simulink model "GlucoseModel2016b"  (R2016b)
settings: Solver=ode4  StartTime=0.0  StopTime=371  FixedStep=.1  RelTol=1e-3  EnableMultiTasking=on
values from neighbouring files (symbols this model uses):
  Bio = min(sqrt(120*12)*rand() + 50, 87) / 100    [GlucoseModelInit.m]
  EGP_0 = lognrnd(log(.0169), .86) * kg    [GlucoseModelInit.m]
  Fs_01 = 11.1 * 10^-3 * kg    (= 0.999)    [GlucoseModelInit.m]
  G_1_0 = 0    [GlucoseModelInit.m]
  G_2_0 = 0    [GlucoseModelInit.m]
  I_0 = 1.15    [GlucoseModelInit.m]
  k_12 = max(min(lognrnd(-2.813, .43), .2), .01)    [GlucoseModelInit.m]
  k_a = max(min(normrnd(.018, .0045), .06), .005)    [GlucoseModelInit.m]
  k_a_int = lognrnd(-2.372, 1.092)    [GlucoseModelInit.m]
  k_b1 = max(min(lognrnd(-5.684, 1.00), .05), .0002)    [GlucoseModelInit.m]
  k_b2 = max(min(lognrnd(-2.882, .75), .4), .005)    [GlucoseModelInit.m]
  k_b3 = max(min(lognrnd(-3.730, .75), .1), .003)    [GlucoseModelInit.m]
  k_e = max(min(normrnd(.14, .0345), .3), .05)    [GlucoseModelInit.m]
  Q_1_0 = G_0 * V_G    (= 203.51601)    [GlucoseModelInit.m]
  R_cl = max(min(normrnd(.01, .025), .03), .003)    [GlucoseModelInit.m]
  R_thr = max(min(normrnd(9, 1.5), 15.0), 7.5)    [GlucoseModelInit.m]
  S_1_0 = 0    [GlucoseModelInit.m]
  S_2_0 = 0    [GlucoseModelInit.m]
  S_ID = 1.58 * 10^-4    (= 0.000158)    [GlucoseModelInit.m]
  S_IE = 73 * 10^-4    (= 0.0073)    [GlucoseModelInit.m]
  S_IT = 11.0 * 10^-4    (= 0.0011)    [GlucoseModelInit.m]
  t_max = 1 / max(min(lognrnd(-3.689, 0.252), .035), .02)    [GlucoseModelInit.m]
  V_G = max(min(lognrnd(-1.897, .23), .25), .09) * kg    [GlucoseModelInit.m]
  V_I = max(min(normrnd(.12, .012), .18), .08) * kg    [GlucoseModelInit.m]
settings Model: Creator=brier245  LastModifiedBy=aegawe01
settings SolverCC: ZeroCrossControl=DisableAll
settings DataIOCC: SaveFormat=Structure  ReturnWorkspaceOutputs=on  ReturnWorkspaceOutputsName=SDOSimTest_Log
settings OptimizationCC: LifeSpan=inf
settings DebuggingCC: SFUnexpectedBacktrackingDiag=warning  SFNoUnconditionalDefaultTransitionDiag=warning  SFExecutionAtInitializationDiag=none
settings HardwareCC: ProdBitPerPointer=32  ProdBitPerSizeT=32  ProdBitPerPtrDiffT=32  ProdLargestAtomicFloat=None  ProdIntDivRoundTo=Undefined  ProdEndianess=Unspecified  ProdWordSize=32  ProdHWDeviceType=32-bit Generic
settings ModelReferenceCC: PropagateSignalLabelsOutOfModel=off
settings GRTTargetCC: TargetLangStandard=C89/C90 (ANSI)  GeneratePreprocessorConditionals=Disable all
settings ConfigComp: CovMetricSettings=dw  CovHtmlReporting=on  CovSaveCumulativeToWorkspaceVar=on  CovSaveSingleToWorkspaceVar=on  CovExternalEMLEnable=off

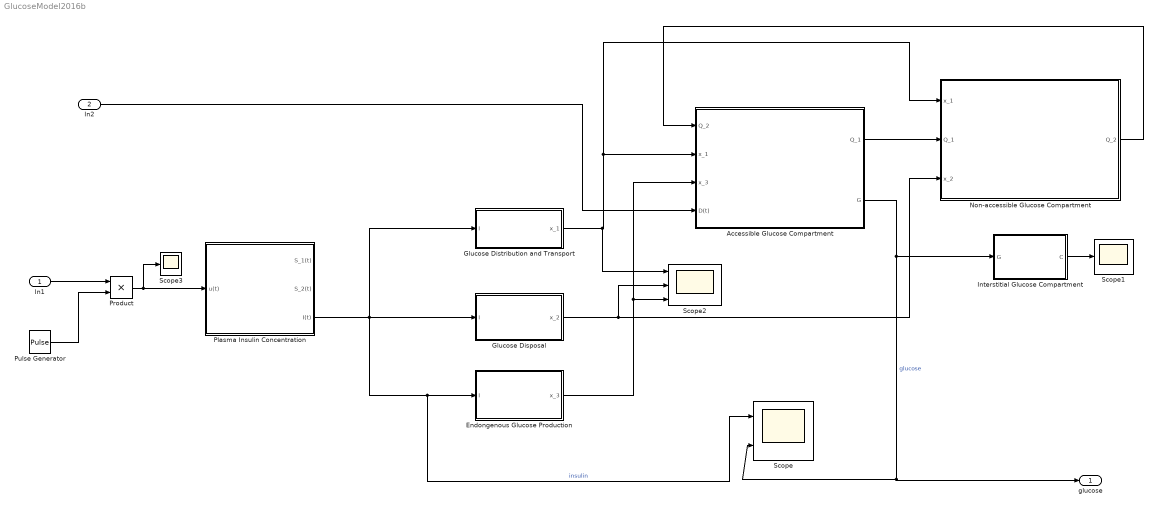
== system GlucoseModel2016b ==
  In1 : Inport
  In2 : Inport  Port=2
  Accessible Glucose Compartment : Subsystem
  Endongenous Glucose Production : Subsystem
  Glucose Disposal : Subsystem
  Glucose Distribution and Transport : Subsystem
  Interstitial Glucose Compartment : Subsystem
  Non-accessible Glucose Compartment : Subsystem
  Plasma Insulin Concentration : Subsystem
  Product : Product
  Pulse Generator : DiscretePulseGenerator  PulseType=Time based  Period=60  PulseWidth=100./60
  Scope : Scope  NumInputPorts=2
  Scope1 : Scope
  Scope2 : Scope  NumInputPorts=3
  Scope3 : Scope
  glucose : Outport
  wires:
  Accessible Glucose Compartment/1(Q_1) -> Non-accessible Glucose Compartment/2(Q_1)
  Non-accessible Glucose Compartment/1(Q_2) -> Accessible Glucose Compartment/1(Q_2)
  Plasma Insulin Concentration/3(I(t)) -> Glucose Distribution and Transport/1(I), Glucose Disposal/1(I), Scope/1, Endongenous Glucose Production/1(I)  "insulin"
  Glucose Distribution and Transport/1(x_1) -> Scope2/1, Accessible Glucose Compartment/2(x_1), Non-accessible Glucose Compartment/1(x_1)
  Glucose Disposal/1(x_2) -> Scope2/2, Non-accessible Glucose Compartment/3(x_2)
  Endongenous Glucose Production/1(x_3) -> Accessible Glucose Compartment/3(x_3), Scope2/3
  Accessible Glucose Compartment/2(G) -> glucose/1, Scope/2, Interstitial Glucose Compartment/1(G)  "glucose"
  Interstitial Glucose Compartment/1(C) -> Scope1/1
  In2/1 -> Accessible Glucose Compartment/4(D(t))
  In1/1 -> Product/1
  Pulse Generator/1 -> Product/2
  Product/1 -> Scope3/1, Plasma Insulin Concentration/1(u(t))

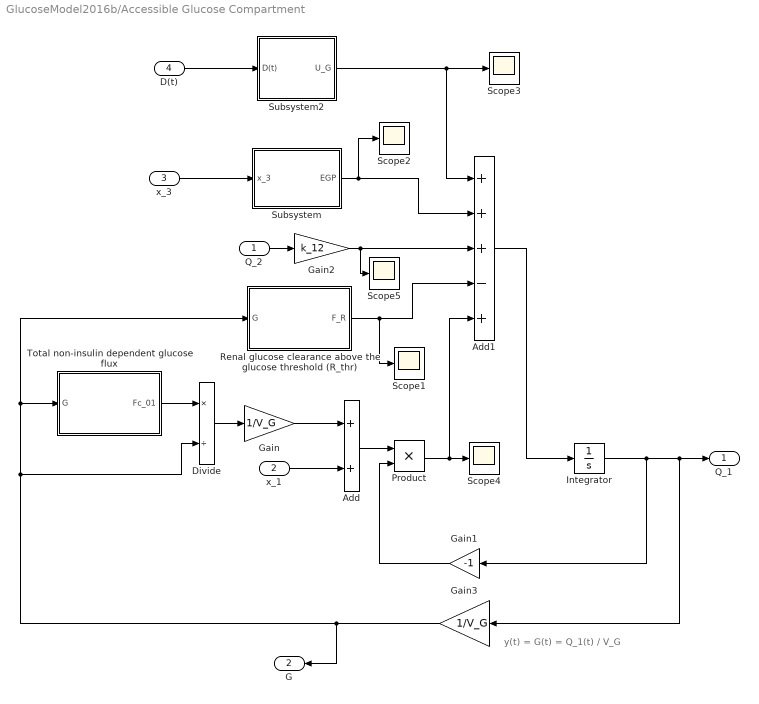
== system GlucoseModel2016b/Accessible Glucose Compartment ==
  note: y(t) = G(t) = Q_1(t) / V_G
  Q_2 : Inport
  x_1 : Inport  Port=2
  x_3 : Inport  Port=3
  D(t) : Inport  Port=4
  Add : Sum
  Add1 : Sum  Inputs=+++-+
  Divide : Product  Inputs=*/
  Gain : Gain  Gain=1/V_G
  Gain1 : Gain  Gain=-1
  Gain2 : Gain  Gain=k_12
  Gain3 : Gain  Gain=1/V_G
  Integrator : Integrator  InitialCondition=Q_1_0  LimitOutput=on  LowerSaturationLimit=0
  Product : Product
  Renal glucose clearance above the glucose threshold (R_thr) : Subsystem
  Scope{1..5} (5 alike) : Scope
  Subsystem : Subsystem
  Subsystem2 : Subsystem
  Total non-insulin dependent glucose flux : Subsystem
  Q_1 : Outport
  G : Outport  Port=2
  wires:
  x_1/1 -> Add/2
  Q_2/1 -> Gain2/1
  Product/1 -> Scope4/1, Add1/5
  Total non-insulin dependent glucose flux/1(Fc_01) -> Divide/1
  Divide/1 -> Gain/1
  Integrator/1 -> Gain3/1, Q_1/1, Gain1/1
  Add1/1 -> Integrator/1
  x_3/1 -> Subsystem/1(x_3)
  Gain1/1 -> Product/2
  Renal glucose clearance above the glucose threshold (R_thr)/1(F_R) -> Scope1/1, Add1/4
  Subsystem/1(EGP) -> Scope2/1, Add1/2
  Gain/1 -> Add/1
  Add/1 -> Product/1
  Gain2/1 -> Scope5/1, Add1/3
  D(t)/1 -> Subsystem2/1(D(t))
  Subsystem2/1(U_G) -> Add1/1, Scope3/1
  Gain3/1 -> G/1, Divide/2, Renal glucose clearance above the glucose threshold (R_thr)/1(G), Total non-insulin dependent glucose flux/1(G)

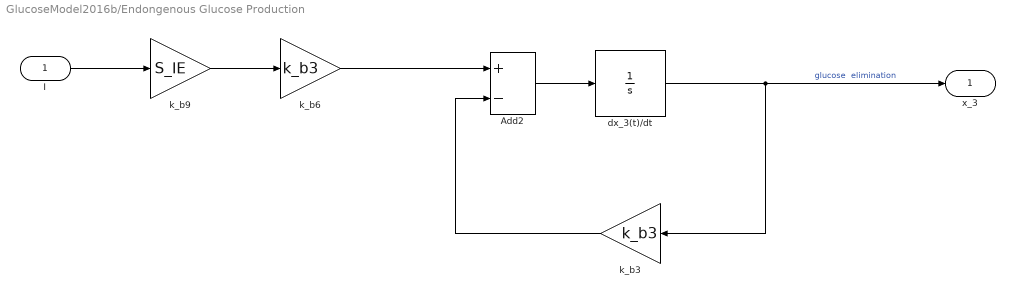
== system GlucoseModel2016b/Endongenous Glucose Production ==
  I : Inport
  Add2 : Sum  Inputs=+-
  dx_3(t)/dt : Integrator  InitialCondition=S_IE*I_0  LimitOutput=on  LowerSaturationLimit=0
  k_b3 : Gain  Gain=k_b3
  k_b6 : Gain  Gain=k_b3
  k_b9 : Gain  Gain=S_IE
  x_3 : Outport
  wires:
  k_b9/1 -> k_b6/1
  dx_3(t)/dt/1 -> x_3/1, k_b3/1  "glucose  elimination"
  Add2/1 -> dx_3(t)/dt/1
  k_b3/1 -> Add2/2
  k_b6/1 -> Add2/1
  I/1 -> k_b9/1

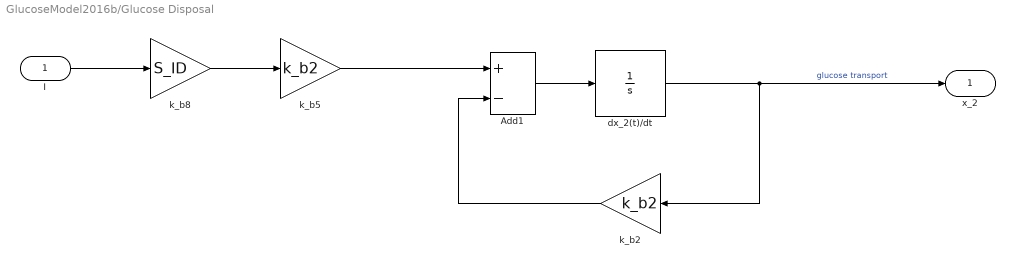
== system GlucoseModel2016b/Glucose Disposal ==
  I : Inport
  Add1 : Sum  Inputs=+-
  dx_2(t)/dt : Integrator  InitialCondition=S_ID*I_0  LimitOutput=on  LowerSaturationLimit=0
  k_b2 : Gain  Gain=k_b2
  k_b5 : Gain  Gain=k_b2
  k_b8 : Gain  Gain=S_ID
  x_2 : Outport
  wires:
  I/1 -> k_b8/1
  dx_2(t)/dt/1 -> x_2/1, k_b2/1  "glucose transport"
  k_b2/1 -> Add1/2
  Add1/1 -> dx_2(t)/dt/1
  k_b5/1 -> Add1/1
  k_b8/1 -> k_b5/1

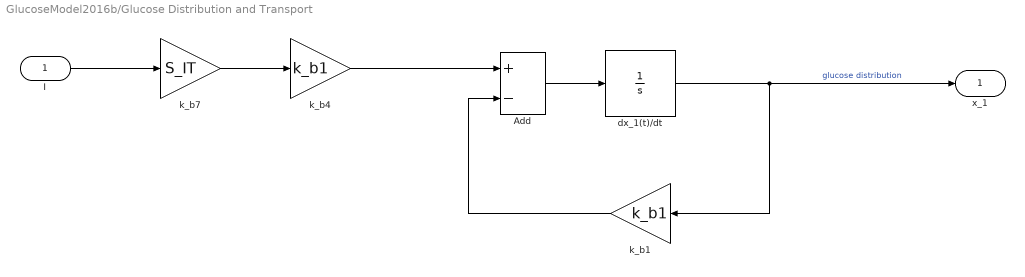
== system GlucoseModel2016b/Glucose Distribution and Transport ==
  I : Inport
  Add : Sum  Inputs=+-
  dx_1(t)/dt : Integrator  InitialCondition=S_IT*I_0  LimitOutput=on  LowerSaturationLimit=0
  k_b1 : Gain  Gain=k_b1
  k_b4 : Gain  Gain=k_b1
  k_b7 : Gain  Gain=S_IT
  x_1 : Outport
  wires:
  I/1 -> k_b7/1
  Add/1 -> dx_1(t)/dt/1
  k_b4/1 -> Add/1
  dx_1(t)/dt/1 -> x_1/1, k_b1/1  "glucose distribution"
  k_b1/1 -> Add/2
  k_b7/1 -> k_b4/1

== system GlucoseModel2016b/Interstitial Glucose Compartment ==
  G : Inport
  Gain : Gain  Gain=k_a_int
  Integrator : Integrator
  Subtract : Sum  Inputs=+-
  C : Outport
  wires:
  G/1 -> Subtract/1
  Subtract/1 -> Gain/1
  Gain/1 -> Integrator/1
  Integrator/1 -> C/1, Subtract/2

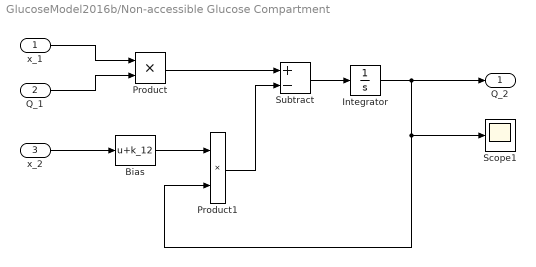
== system GlucoseModel2016b/Non-accessible Glucose Compartment ==
  x_1 : Inport
  Q_1 : Inport  Port=2
  x_2 : Inport  Port=3
  Bias : Bias  Bias=k_12
  Integrator : Integrator  LimitOutput=on  LowerSaturationLimit=0
  Product : Product
  Product1 : Product
  Scope1 : Scope
  Subtract : Sum  Inputs=+-
  Q_2 : Outport
  wires:
  Integrator/1 -> Product1/2, Scope1/1, Q_2/1
  Product/1 -> Subtract/1
  Product1/1 -> Subtract/2
  x_1/1 -> Product/1
  Q_1/1 -> Product/2
  x_2/1 -> Bias/1
  Bias/1 -> Product1/1
  Subtract/1 -> Integrator/1

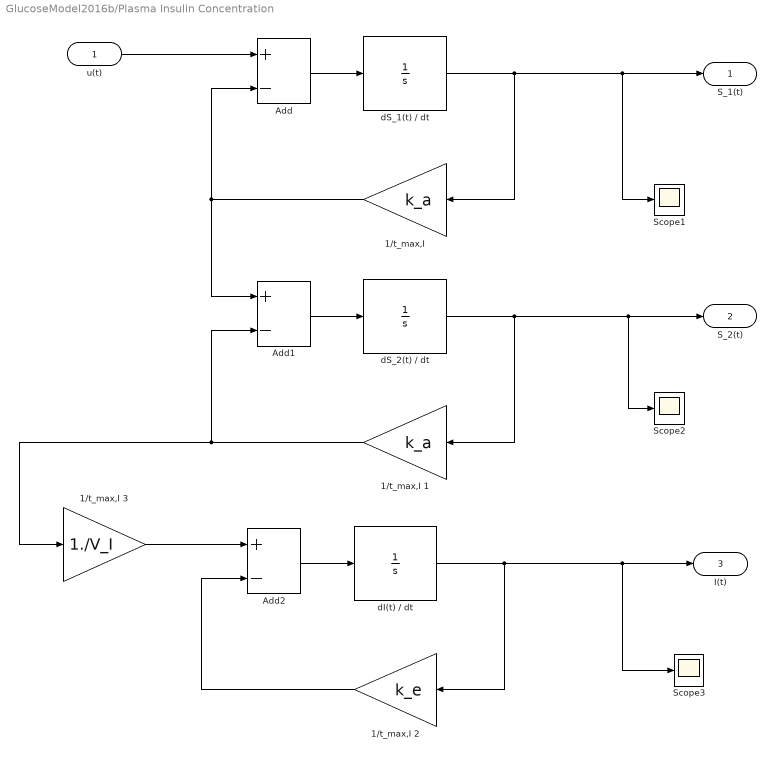
== system GlucoseModel2016b/Plasma Insulin Concentration ==
  u(t) : Inport
  "1/t_max,I " : Gain  Gain=k_a
  1/t_max,I 1 : Gain  Gain=k_a
  1/t_max,I 2 : Gain  Gain=k_e
  1/t_max,I 3 : Gain  Gain=1./V_I
  Add : Sum  Inputs=+-
  Add1 : Sum  Inputs=+-
  Add2 : Sum  Inputs=+-
  Scope1 : Scope
  Scope2 : Scope
  Scope3 : Scope
  dI(t) / dt : Integrator  InitialCondition=I_0  LimitOutput=on  LowerSaturationLimit=0
  dS_1(t) / dt : Integrator  InitialCondition=S_1_0  LimitOutput=on  LowerSaturationLimit=0
  dS_2(t) / dt : Integrator  InitialCondition=S_2_0  LimitOutput=on  LowerSaturationLimit=0
  S_1(t) : Outport
  S_2(t) : Outport  Port=2
  I(t) : Outport  Port=3
  wires:
  "1/t_max,I "/1 -> Add1/1, Add/2
  u(t)/1 -> Add/1
  dS_2(t) / dt/1 -> Scope2/1, S_2(t)/1, 1/t_max,I 1/1
  Add1/1 -> dS_2(t) / dt/1
  dS_1(t) / dt/1 -> Scope1/1, S_1(t)/1, "1/t_max,I "/1
  dI(t) / dt/1 -> Scope3/1, I(t)/1, 1/t_max,I 2/1
  Add2/1 -> dI(t) / dt/1
  1/t_max,I 2/1 -> Add2/2
  1/t_max,I 3/1 -> Add2/1
  1/t_max,I 1/1 -> 1/t_max,I 3/1, Add1/2
  Add/1 -> dS_1(t) / dt/1

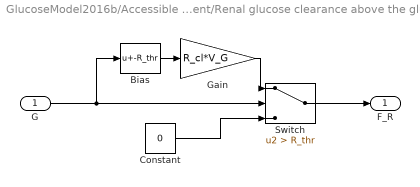
== system GlucoseModel2016b/Accessible Glucose Compartment/Renal glucose clearance above the glucose threshold (R_thr) ==
  G : Inport
  Bias : Bias  Bias=-R_thr
  Constant : Constant  Value=0
  Gain : Gain  Gain=R_cl*V_G
  Switch : Switch  Criteria=u2 > Threshold  Threshold=R_thr
  F_R : Outport
  wires:
  Gain/1 -> Switch/1
  Bias/1 -> Gain/1
  Constant/1 -> Switch/3
  Switch/1 -> F_R/1
  G/1 -> Bias/1, Switch/2

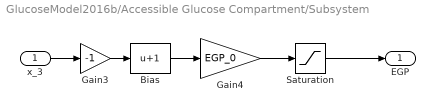
== system GlucoseModel2016b/Accessible Glucose Compartment/Subsystem ==
  x_3 : Inport
  Bias : Bias  Bias=1
  Gain3 : Gain  Gain=-1
  Gain4 : Gain  Gain=EGP_0
  Saturation : Saturate  UpperLimit=inf  LowerLimit=0
  EGP : Outport
  wires:
  x_3/1 -> Gain3/1
  Bias/1 -> Gain4/1
  Gain3/1 -> Bias/1
  Gain4/1 -> Saturation/1
  Saturation/1 -> EGP/1

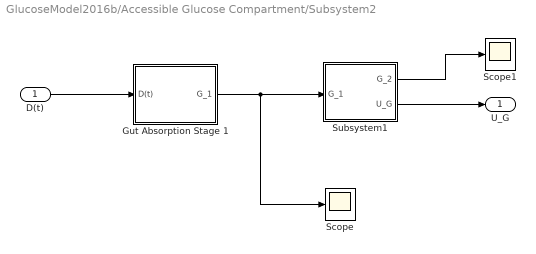
== system GlucoseModel2016b/Accessible Glucose Compartment/Subsystem2 ==
  D(t) : Inport
  Gut Absorption Stage 1 : Subsystem
  Scope : Scope
  Scope1 : Scope
  Subsystem1 : Subsystem
  U_G : Outport
  wires:
  Subsystem1/2(U_G) -> U_G/1
  Gut Absorption Stage 1/1(G_1) -> Scope/1, Subsystem1/1(G_1)
  Subsystem1/1(G_2) -> Scope1/1
  D(t)/1 -> Gut Absorption Stage 1/1(D(t))

== system GlucoseModel2016b/Accessible Glucose Compartment/Total non-insulin dependent glucose flux ==
  G : Inport
  Bias : Bias  Bias=1
  Gain : Gain  Gain=Fs_01
  Product : Product  Inputs=*/
  Fc_01 : Outport
  wires:
  Gain/1 -> Fc_01/1
  G/1 -> Bias/1, Product/1
  Bias/1 -> Product/2
  Product/1 -> Gain/1

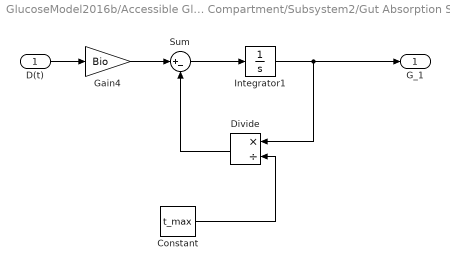
== system GlucoseModel2016b/Accessible Glucose Compartment/Subsystem2/Gut Absorption Stage 1 ==
  D(t) : Inport
  Constant : Constant  Value=t_max
  Divide : Product  Inputs=*/
  Gain4 : Gain  Gain=Bio
  Integrator1 : Integrator  InitialCondition=G_1_0
  Sum : Sum  Inputs=|+-
  G_1 : Outport
  wires:
  D(t)/1 -> Gain4/1
  Gain4/1 -> Sum/1
  Sum/1 -> Integrator1/1
  Integrator1/1 -> Divide/1, G_1/1
  Divide/1 -> Sum/2
  Constant/1 -> Divide/2

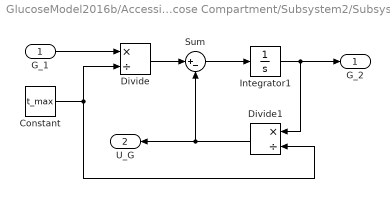
== system GlucoseModel2016b/Accessible Glucose Compartment/Subsystem2/Subsystem1 ==
  G_1 : Inport
  Constant : Constant  Value=t_max
  Divide : Product  Inputs=*/
  Divide1 : Product  Inputs=*/
  Integrator1 : Integrator  InitialCondition=G_2_0
  Sum : Sum  Inputs=|+-
  G_2 : Outport
  U_G : Outport  Port=2
  wires:
  Divide/1 -> Sum/1
  Sum/1 -> Integrator1/1
  Divide1/1 -> U_G/1, Sum/2
  Integrator1/1 -> G_2/1, Divide1/1
  Constant/1 -> Divide1/2, Divide/2
  G_1/1 -> Divide/1
